simulink model "Pratica2_PD_simulink"  (R2020a)
settings: Solver=VariableStepAuto  StartTime=0.0  StopTime=50  RelTol=1e-3
libraries: dspsrcs4 x2
settings Model: Creator=gusta  LastModifiedBy=gusta

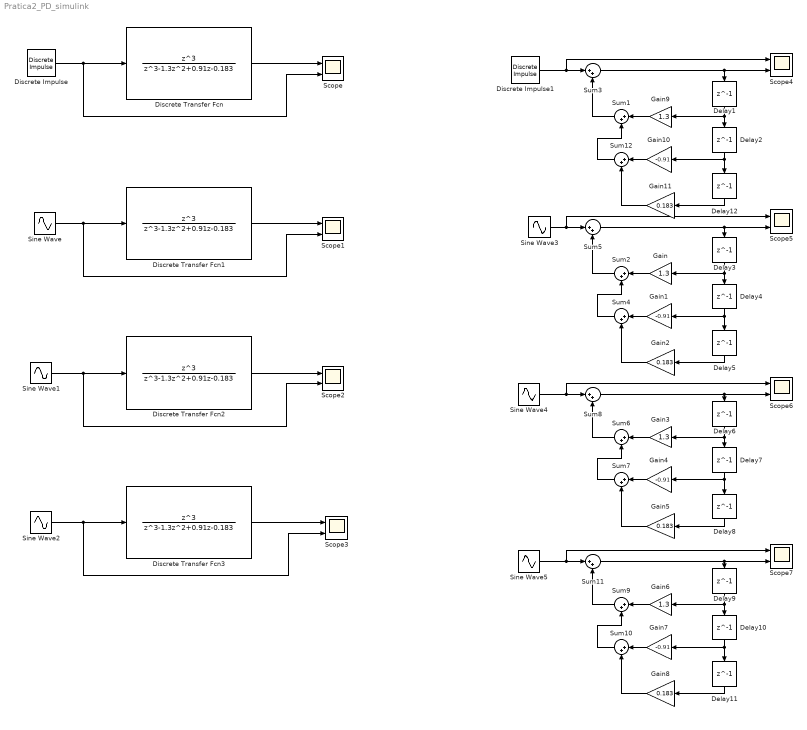
== system Pratica2_PD_simulink ==
  Delay{1..12} (12 alike) : Delay  DelayLength=1
  Discrete Transfer Fcn{,1..3} (4 alike) : DiscreteTransferFcn  Numerator=[1 0 0 0]  Denominator=[1 -1.3 0.91 -0.183]
  Discrete Impulse : dspsrcs4/Discrete  Impulse  Delay=0  SampleTime=1  FrameSample=1  OutputFrames=off  dataType=double  isSigned=on  wordLen=16  udDataType=sfix(16)  fracBitsMode=Best precision  numFracBits=15  OutDataTypeStr=double  LastOutDataTypeStr=double
  Discrete Impulse1 : dspsrcs4/Discrete  Impulse  Delay=0  SampleTime=1  FrameSample=1  OutputFrames=off  dataType=double  isSigned=on  wordLen=16  udDataType=sfix(16)  fracBitsMode=Best precision  numFracBits=15  OutDataTypeStr=double  LastOutDataTypeStr=double
  Gain{,3,6,9} (4 alike) : Gain  Gain=1.3
  Gain{1,4,7,10} (4 alike) : Gain  Gain=-0.91
  Gain{2,5,8,11} (4 alike) : Gain  Gain=0.183
  Scope{,1..7} (8 alike) : Scope  NumInputPorts=2
  Sine Wave : Sin  Frequency=pi/4  SampleTime=0
  Sine Wave1 : Sin  Frequency=pi/2  SampleTime=0
  Sine Wave2 : Sin  Frequency=3*pi/4  SampleTime=0
  Sine Wave3 : Sin  Frequency=pi/4  SampleTime=0
  Sine Wave4 : Sin  Frequency=pi/2  SampleTime=0
  Sine Wave5 : Sin  Frequency=3*pi/4  SampleTime=0
  Sum{1..12} (12 alike) : Sum  Inputs=|++
  wires:
  Discrete Transfer Fcn/1 -> Scope/1
  Discrete Impulse/1 -> Scope/2, Discrete Transfer Fcn/1
  Discrete Transfer Fcn1/1 -> Scope1/1
  Sine Wave/1 -> Scope1/2, Discrete Transfer Fcn1/1
  Discrete Transfer Fcn2/1 -> Scope2/1
  Sine Wave1/1 -> Scope2/2, Discrete Transfer Fcn2/1
  Sine Wave2/1 -> Scope3/2, Discrete Transfer Fcn3/1
  Discrete Transfer Fcn3/1 -> Scope3/1
  Discrete Impulse1/1 -> Scope4/1, Sum3/1
  Sum5/1 -> Delay3/1, Scope5/2
  Sum2/1 -> Sum5/2
  Sum4/1 -> Sum2/2
  Sine Wave3/1 -> Scope5/1, Sum5/1
  Sine Wave4/1 -> Scope6/1, Sum8/1
  Sine Wave5/1 -> Scope7/1, Sum11/1
  Delay5/1 -> Gain2/1
  Gain2/1 -> Sum4/2
  Gain1/1 -> Sum4/1
  Delay4/1 -> Delay5/1, Gain1/1
  Gain/1 -> Sum2/1
  Sum8/1 -> Delay6/1, Scope6/2
  Sum11/1 -> Delay9/1, Scope7/2
  Sum3/1 -> Delay1/1, Scope4/2
  Delay3/1 -> Delay4/1, Gain/1
  Gain9/1 -> Sum1/1
  Gain11/1 -> Sum12/2
  Delay12/1 -> Gain11/1
  Sum1/1 -> Sum3/2
  Delay2/1 -> Delay12/1, Gain10/1
  Delay1/1 -> Delay2/1, Gain9/1
  Gain10/1 -> Sum12/1
  Sum12/1 -> Sum1/2
  Gain3/1 -> Sum6/1
  Gain5/1 -> Sum7/2
  Delay8/1 -> Gain5/1
  Sum6/1 -> Sum8/2
  Delay7/1 -> Delay8/1, Gain4/1
  Delay6/1 -> Delay7/1, Gain3/1
  Gain4/1 -> Sum7/1
  Sum7/1 -> Sum6/2
  Gain6/1 -> Sum9/1
  Gain8/1 -> Sum10/2
  Delay11/1 -> Gain8/1
  Sum9/1 -> Sum11/2
  Delay10/1 -> Delay11/1, Gain7/1
  Delay9/1 -> Delay10/1, Gain6/1
  Gain7/1 -> Sum10/1
  Sum10/1 -> Sum9/2
